simulink model "Lab_04_MinimizingtheTransmissionLossingPowerSystemwitTransformer"  (R2024b)
settings: Solver=VariableStepAuto  StartTime=0.0  StopTime=1  RelTol=1e-3
undefined symbols (not defined in the file): Angle, Magnitude
libraries: spsSeriesRLCBranchLib x4, spsVoltageMeasurementLib x4, spsCurrentMeasurementLib x4, spsLinearTransformerLib x2, spsACVoltageSourceLib x2, sps_lib x1
settings Model: Creator=yashr  LastModifiedBy=yashr

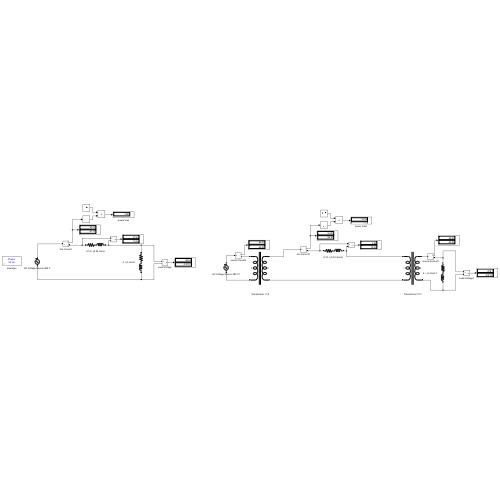
[thumbnail: Simulink's stored preview of the top-level diagram]
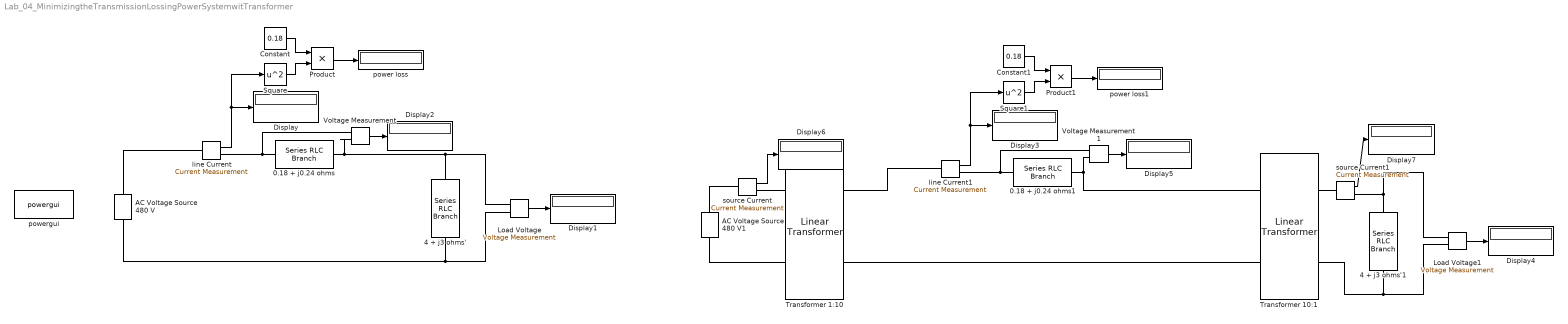
== system Lab_04_MinimizingtheTransmissionLossingPowerSystemwitTransformer ==
  " Transformer 10:1" : spsLinearTransformerLib/Linear Transformer  UNITS=SI  NominalPower=[ 250e6 50]  winding1=[4800 0.0000001 0.0000001]  winding2=[480 0.0000001 0.0000001]  ThreeWindings=off  winding3=[3.15e+05 0.7938 0.084225]  RmLm=[1.0804e+06 2866]  Measurements=None  DataType=on
  " Transformer 1:10" : spsLinearTransformerLib/Linear Transformer  UNITS=SI  NominalPower=[ 250e6 50]  winding1=[480 0.0000001 0.0000001]  winding2=[4800 0.0000001 0.0000001]  ThreeWindings=off  winding3=[3.15e+05 0.7938 0.084225]  RmLm=[1.0804e+06 2866]  Measurements=None  DataType=on
  0.18 + j0.24 ohms : spsSeriesRLCBranchLib/Series RLC Branch  LConnTagsString=__new0  RConnTagsString=__new0  BranchType=RL  Resistance=0.18  Inductance=0.24/(2*pi*50)  SetiL0=off  InitialCurrent=0  Capacitance=1e-6  Setx0=off  InitialVoltage=0  Measurements=None
  0.18 + j0.24 ohms1 : spsSeriesRLCBranchLib/Series RLC Branch  LConnTagsString=__new0  RConnTagsString=__new0  BranchType=RL  Resistance=0.18  Inductance=0.24/(2*pi*50)  SetiL0=off  InitialCurrent=0  Capacitance=1e-6  Setx0=off  InitialVoltage=0  Measurements=None
  4 + j3 ohms' : spsSeriesRLCBranchLib/Series RLC Branch  LConnTagsString=__new0  RConnTagsString=__new0  BranchType=RL  Resistance=4  Inductance=3/(2*pi*50)  SetiL0=off  InitialCurrent=0  Capacitance=1e-6  Setx0=off  InitialVoltage=0  Measurements=None
  4 + j3 ohms'1 : spsSeriesRLCBranchLib/Series RLC Branch  LConnTagsString=__new0  RConnTagsString=__new0  BranchType=RL  Resistance=4  Inductance=3/(2*pi*50)  SetiL0=off  InitialCurrent=0  Capacitance=1e-6  Setx0=off  InitialVoltage=0  Measurements=None
  AC Voltage Source 480 V : spsACVoltageSourceLib/AC Voltage Source  Amplitude=480  Phase=0  Frequency=50  SampleTime=0  Measurements=None  BusType=swing  Pref=10e3  Qref=0  Qmin=-inf  Qmax=+inf
  AC Voltage Source 480 V1 : spsACVoltageSourceLib/AC Voltage Source  Amplitude=480  Phase=0  Frequency=50  SampleTime=0  Measurements=None  BusType=swing  Pref=10e3  Qref=0  Qmin=-inf  Qmax=+inf
  Constant : Constant  Value=0.18
  Constant1 : Constant  Value=0.18
  Display{,1..7} (8 alike) : Display
  Load Voltage : spsVoltageMeasurementLib/Voltage Measurement  PhasorSimulation=on  OutputType=Magnitude-Angle  PSBequivalent=0
  Load Voltage1 : spsVoltageMeasurementLib/Voltage Measurement  PhasorSimulation=on  OutputType=Magnitude-Angle  PSBequivalent=0
  Product : Product
  Product1 : Product
  Square : Math  Operator=square
  Square1 : Math  Operator=square
  Voltage Measurement : spsVoltageMeasurementLib/Voltage Measurement  PhasorSimulation=on  OutputType=Magnitude-Angle  PSBequivalent=0
  Voltage Measurement1 : spsVoltageMeasurementLib/Voltage Measurement  PhasorSimulation=on  OutputType=Magnitude-Angle  PSBequivalent=0
  line Current : spsCurrentMeasurementLib/Current Measurement  PhasorSimulation=on  OutputType=Magnitude-Angle  PSBequivalent=0
  line Current1 : spsCurrentMeasurementLib/Current Measurement  PhasorSimulation=on  OutputType=Magnitude-Angle  PSBequivalent=0
  power loss : Display
  power loss1 : Display
  powergui : sps_lib/powergui  Priority=1  SimulationMode=Phasor  SampleTime=50e-6  frequency=50  Iterations=50  frequencyindice=50  Pbase=100e6  ErrMax=1e-4  UnitsV=kV  UnitsW=MW  buscounter=0  FunctionMessages=off  echomessages=off  EnableUseOfTLC=off  CurrentSourceSwitches=off  DisableSnubberDevices=off  DisableRonSwitches=off  DisableVfSwitches=off  DisplayEquations=off  AutomaticDiscreteSolvers=off  SolverType=Tustin/Backward Euler (TBE)  Interpol=off  ExternalGateDelay=off  methode=off  Ts=100  x0status=blocks  SPID=on  SwTol=0  HookPort=off  NonlinearTolerance=1e-4  nMaxIteration=100  ContinueOnMaxIteration=off  RestoreLinks=warning  ResistiveCurrentMeasurement=off  Frange=[0:2:500]  Ylog=off  Xlog=on  ShowGrid=off  save=off  variable=ZData  structure=0  ZoomFFT=off  StartTime=0.0  cycles=1  DisplayStyle=1  fundamental=60  FreqAxis=off  MaxFrequency=1000  frequencyindicesteady=1  RmsSteady=1  display=off
  source Current : spsCurrentMeasurementLib/Current Measurement  PhasorSimulation=on  OutputType=Magnitude-Angle  PSBequivalent=0
  source Current1 : spsCurrentMeasurementLib/Current Measurement  PhasorSimulation=on  OutputType=Magnitude-Angle  PSBequivalent=0
  wires:
  line Current/1 -> Square/1, Display/1
  Load Voltage/1 -> Display1/1
  Constant/1 -> Product/1
  Square/1 -> Product/2
  Product/1 -> power loss/1
  Voltage Measurement/1 -> Display2/1
  Square1/1 -> Product1/2
  Constant1/1 -> Product1/1
  Product1/1 -> power loss1/1
  Load Voltage1/1 -> Display4/1
  Voltage Measurement1/1 -> Display5/1
  line Current1/1 -> Square1/1, Display3/1
  source Current/1 -> Display6/1
  source Current1/1 -> Display7/1
  connections:
  line Current/RConn1 -- Voltage Measurement/LConn1 -- 0.18 + j0.24 ohms/LConn1
  line Current/LConn1 -- AC Voltage Source 480 V/RConn1
  AC Voltage Source 480 V/LConn1 -- Load Voltage/LConn2 -- 4 + j3 ohms'/RConn1
  0.18 + j0.24 ohms/RConn1 -- Voltage Measurement/LConn2 -- 4 + j3 ohms'/LConn1 -- Load Voltage/LConn1
  Load Voltage1/LConn1 -- source Current1/RConn1 -- 4 + j3 ohms'1/LConn1
  Load Voltage1/LConn2 -- " Transformer 10:1"/RConn2 -- 4 + j3 ohms'1/RConn1
  line Current1/RConn1 -- Voltage Measurement1/LConn1 -- 0.18 + j0.24 ohms1/LConn1
  " Transformer 1:10"/RConn1 -- line Current1/LConn1
  AC Voltage Source 480 V1/LConn1 -- " Transformer 1:10"/LConn2
  0.18 + j0.24 ohms1/RConn1 -- " Transformer 10:1"/LConn1 -- Voltage Measurement1/LConn2
  " Transformer 10:1"/LConn2 -- " Transformer 1:10"/RConn2
  source Current/LConn1 -- AC Voltage Source 480 V1/RConn1
  source Current/RConn1 -- " Transformer 1:10"/LConn1
  source Current1/LConn1 -- " Transformer 10:1"/RConn1
